simulink model "csv_viewer"  (R2020a)
settings: Solver=FixedStepDiscrete  StartTime=0.0  StopTime=1500  FixedStep=0.1  RelTol=1e-3
libraries: simulink_extras x1
settings Model: Creator=nao12  LastModifiedBy=nao12
settings DataIOCC: SaveOutput=off  SignalLogging=off  DSMLogging=off  SaveTime=off  ReturnWorkspaceOutputs=off
settings OptimizationCC: DefaultParameterBehavior=Inlined  EnhancedBackFolding=on  PassReuseOutputArgsAs=Individual arguments  OptimizeBlockOrder=speed  DifferentSizesBufferReuse=on  OptimizationCustomize=off  EfficientTunableParamExpr=on
settings DebuggingCC: ParameterTunabilityLossMsg=error  ArithmeticOperatorsInVariantConditions=warning
settings SFSimCC: MATLABDynamicMemAlloc=off  CustomCodeUndefinedFunction=UseInterfaceOnly
settings RTWCC: SystemTargetFile=ert.tlc  GenCodeOnly=on  TemplateMakefile=ert_default_tmf  GenerateReport=on  RTWUseSimCustomCode=on  IncludeHyperlinkInReport=on  LaunchReport=on  GenerateTraceInfo=on  GenerateTraceReport=on  GenerateTraceReportSl=on  GenerateTraceReportSf=on  GenerateTraceReportEml=on
settings CodeAppCC: ForceParamTrailComments=on  IgnoreCustomStorageClasses=off  OperatorAnnotations=on  SimulinkDataObjDesc=on  SFDataObjDesc=on  InsertBlockDesc=on
settings ERTTargetCC: TargetLangStandard=C99 (ISO)  GenerateSampleERTMain=on  InlinedParameterPlacement=NonHierarchical  ERTCustomFileTemplate=example_file_process.tlc  EnableUserReplacementTypes=on

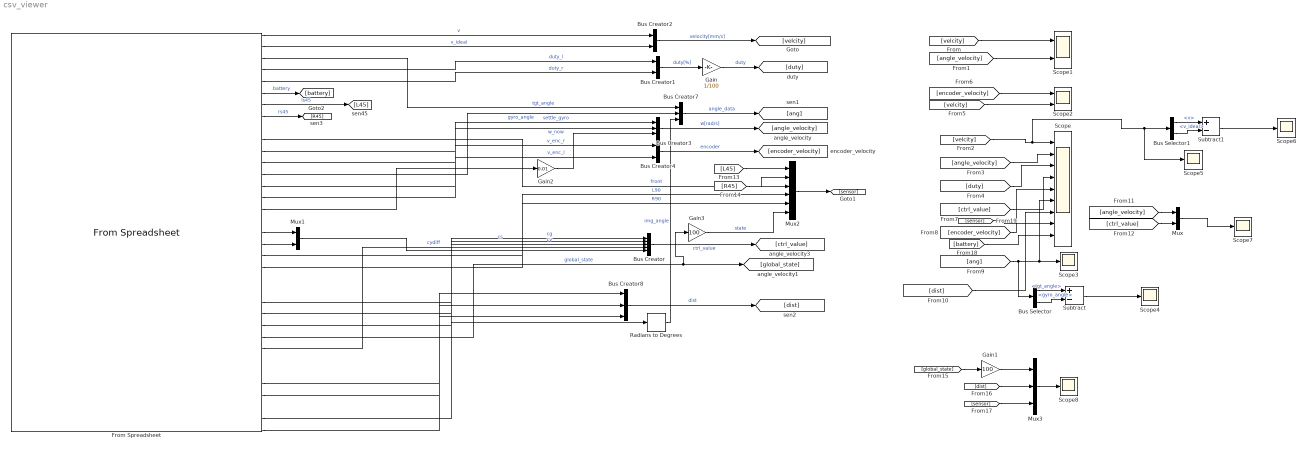
== system csv_viewer ==
  Bus Creator : BusCreator  Inputs=5
  Bus Creator1 : BusCreator  Inputs=2
  Bus Creator2 : BusCreator  Inputs=2
  Bus Creator3 : BusCreator  Inputs=3
  Bus Creator4 : BusCreator  Inputs=2
  Bus Creator7 : BusCreator  Inputs=3
  Bus Creator8 : BusCreator  Inputs=3
  Bus Selector : BusSelector  OutputSignals=tgt_angle,gyro_angle
  Bus Selector1 : BusSelector  OutputSignals=v,v_ideal
  From Spreadsheet : FromSpreadsheet  FileName=test.csv  SheetName=test
  Gain : Gain  Gain=1/100
  Gain1 : Gain  Gain=100
  Gain2 : Gain  Gain=0.01
  Gain3 : Gain  Gain=100
  Mux : Mux  Inputs=2
  Mux1 : Mux  Inputs=2
  Mux2 : Mux  Inputs=6
  Mux3 : Mux  Inputs=3
  Radians to Degrees : simulink_extras/Transformations/Radians to Degrees
  Scope : Scope  NumInputPorts=9
  Scope1 : Scope  NumInputPorts=2
  Scope2 : Scope  NumInputPorts=2
  Scope{3..8} (6 alike) : Scope
  Subtract : Sum  Inputs=+-
  Subtract1 : Sum  Inputs=+-
  wires:
  From Spreadsheet/1 -> Bus Creator2/1  "v"
  From Spreadsheet/2 -> Bus Creator2/2  "v_ideal"
  Bus Creator2/1 -> [velcity]  "velocity[mm/s]"
  From Spreadsheet/11 -> Bus Creator3/1  "settle_gyro"
  From Spreadsheet/12 -> Bus Creator3/2  "w_now"
  Bus Creator3/1 -> [angle_velocity]  "w[rad/s]"
  From Spreadsheet/4 -> Bus Creator1/1  "duty_l"
  From Spreadsheet/5 -> Bus Creator1/2  "duty_r"
  Bus Creator1/1 -> Gain/1  "duty[%]"
  Gain/1 -> [duty]  "duty"
  Bus Creator/1 -> [ctrl_value]  "ctrl_value"
  From Spreadsheet/24 -> Bus Creator/1  "cg"
  From Spreadsheet/25 -> Bus Creator/2  "cs"
  From Spreadsheet/26 -> Bus Creator/3  "cv"
  From Spreadsheet/14 -> Bus Creator4/1  "v_enc_r"
  From Spreadsheet/15 -> Bus Creator4/2  "v_enc_l"
  Bus Creator4/1 -> [encoder_velocity]  "encoder"
  [velcity] -> Scope1/1
  [angle_velocity] -> Scope1/2
  [angle_velocity] -> Scope/2
  [duty] -> Scope/3
  [encoder_velocity] -> Scope2/1
  [velcity] -> Scope2/2
  [ctrl_value] -> Scope/4
  From Spreadsheet/7 -> [L45]  "ls45"
  From Spreadsheet/8 -> [R45]  "rs45"
  From Spreadsheet/20 -> Mux2/4  "L90"
  From Spreadsheet/21 -> Mux2/5  "R90"
  [encoder_velocity] -> Scope/5
  From Spreadsheet/13 -> Bus Creator7/2  "gyro_angle"
  From Spreadsheet/3 -> Bus Creator7/1  "tgt_angle"
  Bus Creator7/1 -> [ang]  "angle_data"
  [ang] -> Bus Selector/1, Scope3/1, Scope/6
  Bus Selector/1 -> Subtract/1  "<tgt_angle>"
  Bus Selector/2 -> Subtract/2  "<gyro_angle>"
  Subtract/1 -> Scope4/1
  Bus Selector1/2 -> Subtract1/2  "<v_ideal>"
  Bus Selector1/1 -> Subtract1/1  "<v>"
  Subtract1/1 -> Scope6/1
  [velcity] -> Scope5/1, Bus Selector1/1, Scope/1
  Bus Creator8/1 -> [dist]  "dist"
  From Spreadsheet/31 -> Bus Creator8/1
  From Spreadsheet/32 -> Bus Creator8/2
  [dist] -> Scope/7
  From Spreadsheet/35 -> Bus Creator8/3
  From Spreadsheet/34 -> Radians to Degrees/1
  Radians to Degrees/1 -> Bus Creator7/3  "img_angle"
  From Spreadsheet/27 -> [global_state], Gain3/1  "global_state"
  From Spreadsheet/16 -> Gain2/1
  From Spreadsheet/28 -> Bus Creator/4  "cydiff"
  Mux/1 -> Scope7/1
  [angle_velocity] -> Mux/1
  [ctrl_value] -> Mux/2
  From Spreadsheet/18 -> Mux1/1
  From Spreadsheet/19 -> Mux1/2
  Mux1/1 -> Bus Creator/5
  From Spreadsheet/10 -> Mux2/3  "front"
  Mux2/1 -> [sensor]
  [L45] -> Mux2/1
  [R45] -> Mux2/2
  [global_state] -> Gain1/1
  Mux3/1 -> Scope8/1
  [dist] -> Mux3/2
  [sensor] -> Mux3/3
  Gain1/1 -> Mux3/1
  Gain2/1 -> Bus Creator3/3
  Gain3/1 -> Mux2/6  "state"
  From Spreadsheet/6 -> [battery]  "battery"
  [battery] -> Scope/9
  [sensor] -> Scope/8
